simulink model "form_filter"  (R2024a)
settings: Solver=VariableStepAuto  StartTime=0.0  StopTime=100  RelTol=1e-8  AbsTol=1e-10
libraries: dspstat3 x4, simulink x3
settings Model: Creator=evgenijkondratev  LastModifiedBy=evgenijkondratev

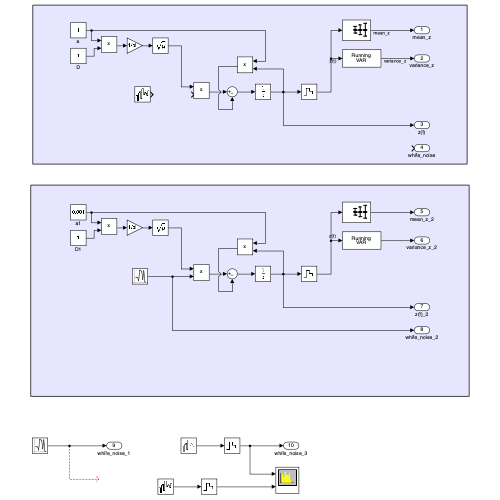
[thumbnail: Simulink's stored preview of the top-level diagram]
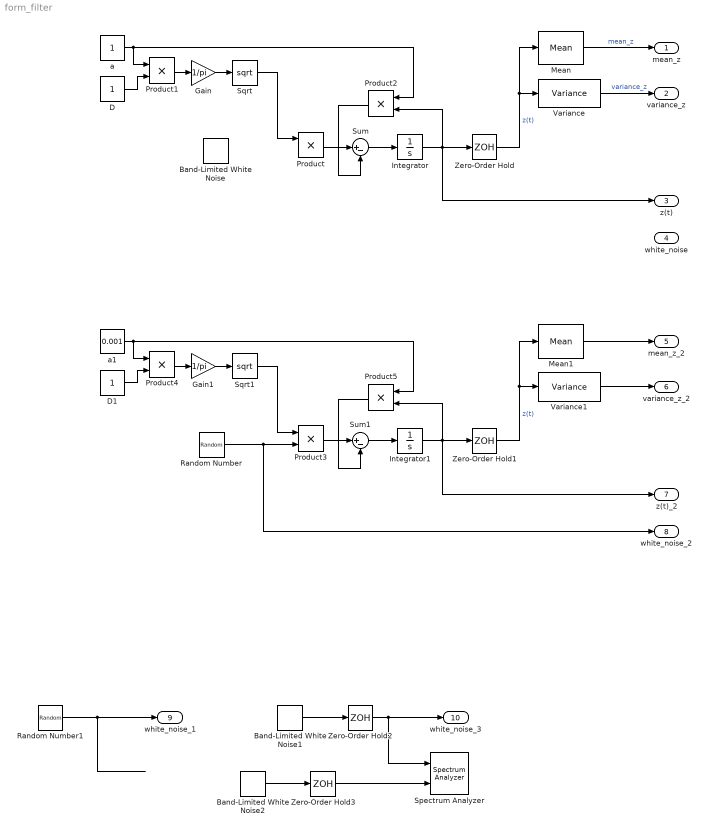
== system form_filter ==
  Band-Limited White Noise : simulink/Sources/Band-Limited White Noise  Cov=[1]  Ts=0.001  seed=[23341]
  Band-Limited White Noise1 : simulink/Sources/Band-Limited White Noise  Cov=[1]  Ts=0.1  seed=[23341]
  Band-Limited White Noise2 : simulink/Sources/Band-Limited White Noise  Cov=[1]  Ts=0.01  seed=[23341]
  D : Constant
  D1 : Constant
  Gain : Gain  Gain=1/pi
  Gain1 : Gain  Gain=1/pi
  Integrator : Integrator
  Integrator1 : Integrator
  Mean : dspstat3/Mean  run=on  reset_popup=None  directionMode=Each column  dimension=1  roiEnable=off  roiType=Rectangles  roiPortion=Entire ROI  roiOutput=Individual statistics for each ROI  roiFlag=off  roundingMode=Floor  overflowMode=off  outputDataTypeStr=Inherit: Same as accumulator  outputMin=[]  outputMax=[]  outputLastDataTypeStr=Inherit: Same as accumulator
  Mean1 : dspstat3/Mean  run=on  reset_popup=None  directionMode=Each column  dimension=1  roiEnable=off  roiType=Rectangles  roiPortion=Entire ROI  roiOutput=Individual statistics for each ROI  roiFlag=off  roundingMode=Floor  overflowMode=off  outputDataTypeStr=Inherit: Same as accumulator  outputMin=[]  outputMax=[]  outputLastDataTypeStr=Inherit: Same as accumulator
  Product{,1..5} (6 alike) : Product
  Random Number : RandomNumber  Variance=10  SampleTime=0.001
  Random Number1 : RandomNumber  Variance=10  SampleTime=0.001
  Spectrum Analyzer : SpectrumAnalyzer  NumInputPorts=2  WindowPosition=[170.000000,173.000000,1565.000000,787.000000,]  ScopeFrameLocation=window  SpectrumType=Power density  SpectrumUnits=dBm/Hz  YLimits=[-37.17822809,37.41095231]
  Sqrt : Sqrt
  Sqrt1 : Sqrt
  Sum : Sum  Inputs=|+-
  Sum1 : Sum  Inputs=|+-
  Variance : dspstat3/Variance  run=on  reset_popup=None  directionMode=Each column  dimension=1  roiEnable=off  roiType=Rectangles  roiPortion=Entire ROI  roiOutput=Individual statistics for each ROI  roiFlag=off  roundingMode=Floor  overflowMode=off
  Variance1 : dspstat3/Variance  run=on  reset_popup=None  directionMode=Each row  dimension=1  roiEnable=off  roiType=Rectangles  roiPortion=Entire ROI  roiOutput=Individual statistics for each ROI  roiFlag=off  roundingMode=Floor  overflowMode=off
  Zero-Order Hold{,1..3} (4 alike) : ZeroOrderHold  SampleTime=0.001
  a : Constant
  a1 : Constant  Value=0.001
  mean_z : Outport
  variance_z : Outport  Port=2
  z(t) : Outport  Port=3
  white_noise : Outport  Port=4
  mean_z_2 : Outport  Port=5
  variance_z_2 : Outport  Port=6
  z(t)_2 : Outport  Port=7
  white_noise_2 : Outport  Port=8
  white_noise_1 : Outport  Port=9
  white_noise_3 : Outport  Port=10
  wires:
  Zero-Order Hold/1 -> Variance/1, Mean/1  "z(t)"
  Integrator/1 -> z(t)/1, Zero-Order Hold/1, Product2/2
  a/1 -> Product2/1, Product1/1
  D/1 -> Product1/2
  Product1/1 -> Gain/1
  Gain/1 -> Sqrt/1
  Sqrt/1 -> Product/1
  Product/1 -> Sum/1
  Product2/1 -> Sum/2
  Sum/1 -> Integrator/1
  Mean/1 -> mean_z/1  "mean_z"
  Variance/1 -> variance_z/1  "variance_z"
  Random Number/1 -> white_noise_2/1, Product3/2
  Gain1/1 -> Sqrt1/1
  Sum1/1 -> Integrator1/1
  Sqrt1/1 -> Product3/1
  Variance1/1 -> variance_z_2/1
  a1/1 -> Product5/1, Product4/1
  Product5/1 -> Sum1/2
  Product4/1 -> Gain1/1
  Zero-Order Hold1/1 -> Variance1/1, Mean1/1  "z(t)"
  Product3/1 -> Sum1/1
  D1/1 -> Product4/2
  Integrator1/1 -> z(t)_2/1, Zero-Order Hold1/1, Product5/2
  Mean1/1 -> mean_z_2/1
  Random Number1/1 -> white_noise_1/1
  Band-Limited White Noise1/1 -> Zero-Order Hold2/1
  Zero-Order Hold2/1 -> Spectrum Analyzer/1, white_noise_3/1
  Band-Limited White Noise2/1 -> Zero-Order Hold3/1
  Zero-Order Hold3/1 -> Spectrum Analyzer/2
